simulink model "TwoRacecars"  (R2022b)
settings: Solver=VariableStepAuto  StartTime=0.0  StopTime=10.0  RelTol=1e-3
values from neighbouring files (symbols this model uses):
  K1 = lqr(A,B,Q1,R1)    [TwoRacecars_init.m]
  K2 = lqr(A,B,Q2,R2)    [TwoRacecars_init.m]
  x0 = 0    [TwoRacecars_init.m]
  xd0 = 0    [TwoRacecars_init.m]
settings Model: Creator=logan  LastModifiedBy=logan

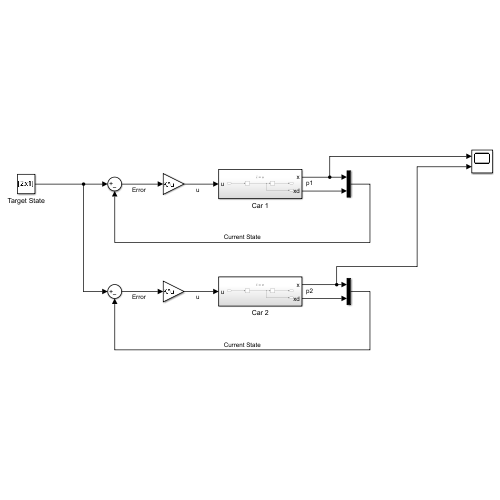
[thumbnail: Simulink's stored preview of the top-level diagram]
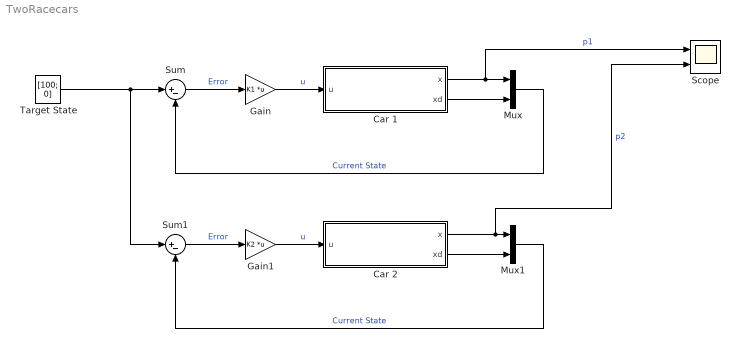
== system TwoRacecars ==
  Car 1 : Subsystem
  Car 2 : Subsystem
  Gain : Gain  Gain=K1  Multiplication=Matrix(K*u)
  Gain1 : Gain  Gain=K2  Multiplication=Matrix(K*u)
  Mux : Mux  Inputs=2
  Mux1 : Mux  Inputs=2
  Scope : Scope  NumInputPorts=2
  Sum : Sum  Inputs=|+-
  Sum1 : Sum  Inputs=|+-
  Target State : Constant  Value=[100; 0]
  wires:
  Car 1/2(xd) -> Mux/2
  Car 1/1(x) -> Scope/1, Mux/1  "p1"
  Mux/1 -> Sum/2  "Current State"
  Sum/1 -> Gain/1  "Error"
  Gain/1 -> Car 1/1(u)  "u"
  Mux1/1 -> Sum1/2  "Current State"
  Target State/1 -> Sum1/1, Sum/1
  Gain1/1 -> Car 2/1(u)  "u"
  Car 2/1(x) -> Scope/2, Mux1/1  "p2"
  Sum1/1 -> Gain1/1  "Error"
  Car 2/2(xd) -> Mux1/2

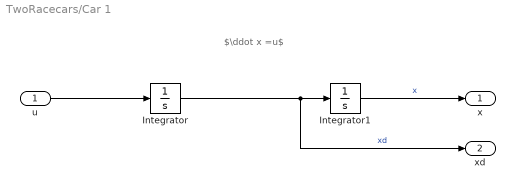
== system TwoRacecars/Car 1 ==
  note: $\ddot x =u$
  u : Inport
  Integrator : Integrator  InitialCondition=xd0
  Integrator1 : Integrator  InitialCondition=x0
  x : Outport
  xd : Outport  Port=2
  wires:
  Integrator/1 -> xd/1, Integrator1/1  "xd"
  Integrator1/1 -> x/1  "x"
  u/1 -> Integrator/1

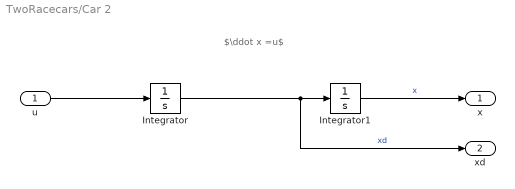
== system TwoRacecars/Car 2 ==
  note: $\ddot x =u$
  u : Inport
  Integrator : Integrator  InitialCondition=xd0
  Integrator1 : Integrator  InitialCondition=x0
  x : Outport
  xd : Outport  Port=2
  wires:
  Integrator/1 -> xd/1, Integrator1/1  "xd"
  Integrator1/1 -> x/1  "x"
  u/1 -> Integrator/1
